simulink model "SML_SSE_RL"  (R2015a)
settings: Solver=ode4  SolverMode=MultiTasking  StartTime=0.0  StopTime=inf  FixedStep=BKIN_STEP_TIME  RelTol=1e-3
StartFcn:
  |  warndlg('Dexterit-E models cannot run under simulation. Please compile your model and run it from within Dexterit-E.');set_param(bdroot,'SimulationCommand','stop')
model workspace (MAT data in the model file):
  col_x = 1
  col_y = 2
  RADIUS_VIS = 3
  COLOR_INIT = 6
  BKIN_STEP_TIME = 0.00025
  E_END_TRIAL = 20
  STROKE_WIDTH = 8
  K_ROBOT_RAMP_TIME = 1
  E_ENABLED_CONTROLLER = 31
  K_TIME_TO_START = 4
  BKIN_KINEMATIC_FRAME_SIZE = 400
  E_NO_EVENT = 0
  STARTTARGET_COL = 1
  MOVE_TIME_COL = 3
  MOVE_XVEL_COL = 4
  MOVE_YVEL_COL = 5
  E_INIT_TRIAL = 1
  E_MOVE_TO_START = 2
  E_AT_START = 4
  E_PASSIVE_HOLD_AT_START = 6
  E_MOVE_TO_END = 8
  COLOR_SELECT = 7
  ACTORPAS_COL = 6
  E_ACTIVE_HOLD_AT_START = 7
  CHANNEL_WIDTH = 1
  WALL_WIDTH = 2
  WALL_STIFFNESS = 3
  WALL_VISCOSITY = 4
  PROBE_COL = 8
  K_TIME_HOLD_START = 5
  E_ENABLE_BUTTONS = 46
  E_DISABLE_BUTTONS = 47
  LABEL_1 = 3
  RESPONSE_AHEAD = 4
  RESPONSE_BEHIND = 5
  B_LABEL_1 = 3
  B_AHEAD = 4
  B_BEHIND = 5
  DYNOREND_COL = 7
  E_REPEAT_TRIAL_FLAG = 35
  END_TARGET_COL = 2
  HEIGHT_VIS = 4
  WIDTH_VIS = 5
  E_TOO_FAST = 11
  E_TOO_SLOW = 12
  PROBE_SHIFT_COL = 9
  K_TIME_PROBE_HOLD = 3
  E_AT_END_TARGET = 10
  K_DELAY_POSTTRIAL = 2
  LABEL_TEXT = 9
  LABEL_HEIGHT = 10
  E_FINISH_MOVE = 49
  E_HIT_PROBE = 48
  E_TEST_1 = 50
  E_JUST_RIGHT = 51
undefined symbols (not defined in the file): slselsubs
libraries: slrtlib x5, KINARM_loads x4, Video x4, General x3, KINARM_general x2, simulink x1, xpcnilib x1
(part 1 of 2)
CloseFcn:
  | rtwprivate ssgencode ModelCloseRequest b2lab2d
settings Model: ModifiedComment=chris -- Wed Feb 16 09:18:30 2005 -- Version 1.1384  ModifiedHistory=Feb 16/05 - Add error repeat, add offset ramp  ExtModeArmWhenConnect=off  ExtModeLogAll=off  Creator=Chris Grebeldinger  LastModifiedBy=User
settings SolverCC: EnableConcurrentExecution=on  AutoInsertRateTranBlk=on
settings DataIOCC: LimitDataPoints=off  SignalLoggingSaveFormat=ModelDataLogs  SaveOutput=off  SaveTime=off  SignalLoggingName=sigsOut
settings OptimizationCC: BlockReduction=off  BooleanDataType=off  OptimizeBlockIOStorage=off  BufferReuse=off  GlobalBufferReuse=off  ExpressionFolding=off  ExpressionDepthLimit=2147483647  LocalBlockOutputs=off  InitFltsAndDblsToZero=on
settings DebuggingCC: SaveWithParameterizedLinksMsg=none  UnderspecifiedInitializationDetection=Classic  MergeDetectMultiDrivingBlocksExec=none  SignalResolutionControl=TryResolveAllWithWarning  MultiTaskDSMMsg=warning  FcnCallInpInsideContextMsg=UseLocalSettings  StateNameClashWarn=warning  StrictBusMsg=ErrorOnBusTreatedAsVector
settings HardwareCC: ProdIntDivRoundTo=Zero  ProdEndianess=LittleEndian  ProdLongLongMode=on  ProdHWDeviceType=Generic->32-bit x86 compatible  TargetHWDeviceType=32-bit Generic
settings SFSimCC: SimCustomHeaderCode="#include \"stdlib.h\""  SFSimEcho=off  SimParseCustomCode=off
settings RTWCC: SystemTargetFile=slrt.tlc  TemplateMakefile=slrt_default_tmf  Description=Simulink Real-Time  CustomSourceCode="#include \"stdlib.h\""
settings CodeAppCC: MaxIdLength=63
settings SimulinkRealTimeCC: TargetFcnLib=ansi_tfl_tmw.mat  GeneratePreprocessorConditionals=Disable all  xPCisDownloadable=off  xPCisDefaultEnv=off

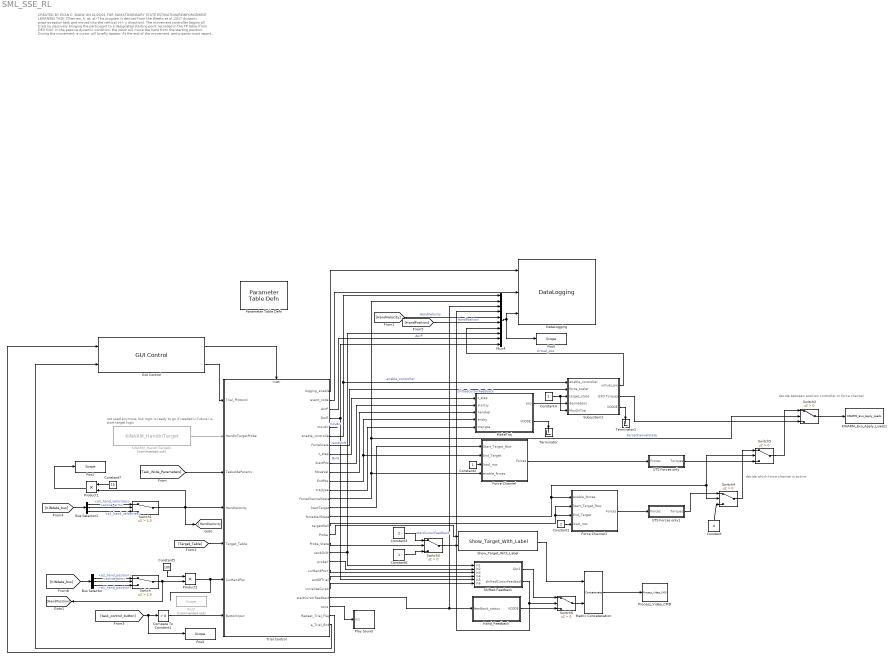
== system SML_SSE_RL ==
  note: not used anymore, but logic is ready to go if needed in future
      | i.e. start target logic
  note: decide between position controller or force channel
  note: decide which force channel is active
  note: CREATED BY EVAN C. SNOW ON 01/25/21 FOR SOMATOSENSORY STATE ESTIMATION/REINFORCEMENT LEARNING TASK (Therrien, A. et. al)
      | This program is derived from the Weeks et al. 2017 dynamic proprioception task and moved into the vertical (+/- y direction). The movement controller begins all trials by passively bringing the participant to a designated starting point recorded in the TP table (from DEX GUI).
      |
      | In the passive dynamic condition, the robot will move the hand from the starting position. During the movement, a cursor will briefly appear. At the end of the movement, participants must report if the cursor was "ahead" or "behind".
      |
      | In the passive endpoint condition, the robot will move the hand from the starting position to a designated probe somewhere between the start and end points (designated by the TP table in DEX GUI). It will then hold the fingertip veridical to the center of the probe and briefly display a cursor. After extinguishing the cursor, the movement controller will move the finger tip from the probe to the end target. At the end of the movement, participants must report if the cursor was "ahead" or "behind".
      |
      | In the active dynamic condition, participants will be held at a start point until a beep sounds, then they begin moving (as instructed). A cursor will appear briefly during the movement. The robot will stop the participant's hand at the end point. The participant must then report if the cursor was "ahead" or "behind". A force channel will enforce movement direction, and behavioral feedback will be used to maintain movement speed.
      |
      | In the active endpoint condition, participants will be held at a start point until a beep sounds, then they begin moving (as instructed). A cursor will appear briefly during the movement. The robot will stop the participant's hand at the y location of the probe and a cursor will briefly display. After extinguishing the cursor, the participant will move the finger tip from the probe to the end target. The participant must then report if the cursor was "ahead" or "behind". A force channel will enforce movement direction, and behavioral feedback will be used to maintain movement speed (behavioral feedback for this section is based on both phases individually i.e. start to probe and probe to end).
      |
      | For all trials, the cursor could be shifted +/- 0, 7, 13, 20, 30, 40 mm. The movement controller constant velocity was set to 0.5 m/s. The cursor was shown veridically before movement for 600 ms and somewhere between the start and endpoint (probe location) for 600 ms with logic depending on each task. The recording of the response from the patient is recorded using Task Buttons and is evident in the DEX GUI.
  Bus Selector : BusSelector  OutputSignals=Robot2.a2_hand_position,KINDataGeneral.active_arm,Robot1.a1_hand_position
  Bus Selector1 : BusSelector  OutputSignals=Robot2.a2_hand_velocities,KINDataGeneral.active_arm,Robot1.a1_hand_velocities
  Compare To Constant1 : simulink/Logic and Bit Operations/Compare To Constant  relop=>  const=0  OutDataTypeStr=boolean
  Constant : Constant  Value=0
  Constant1 : Constant  Value=2
  Constant2 : Constant
  Constant3 : Constant  Value=2
  Constant4 : Constant
  Constant5 : Constant  Value=100
  Constant6 : Constant
  Constant7 : Constant  Value=10
  DataLogging : General/DataLogging  log_event_codes=on  log_analog_inputs=on  show_time_remaining=off  ecat_include=on
  Force Channel : Subsystem
  Force Channel1 : Subsystem
  GUI Control : General/GUI Control  task_version=1.0  show_repeat_trial_flag=on  use_custom_tp=off  target_type_str=Circle  Target_Type=1  XYcols=[1 2]  Vcols=3  Lcols=4  indices_padding=[0 0 0 0;0 0 0 0]  target_table_rows=64  load_table_rows=20  tp_table_rows=100
  Hand_Feedback : Subsystem  AncestorBlock=KINARM_general/Hand_Feedback  mask(Hand_Feedback){feedback_cntl_src=status only}
      mask prompts: feedback_cntl_src "Task Program control of style and status"
      mask help:
      | This block controls various options for hand feedback (i.e. fingertip position)  to be shown to the subject.
      |
      | Task Program control of style and status refers to whether the Program Task will explicity control the style and/or status of the hand feedback.
      mask init:
      | block_path = gcb;  % store block path, as gcb may change with block operations
      | 
      | %%% Handle background colours if link status changes.  
      | checkBackgroundColour(block_path, 'KINARM_general');
      | 
      | 
      | feedback_cntl_source=get_param(gcb,'feedback_cntl_src');
      | 
      | if feedback_cntl_source(1:4)=='none'
      |     block1type='Constant';
      |     block2type='Constant';
      |     block3type='Constant';
      | elseif feedback_cntl_source(1:4)=='stat'
      |     block1type='Constant';
      |     block2type='Constant';
      |     block3type='Inport';
      | else 
      |     block1type='Inport';
      |     block2type='Inport';
      |     block3type='Constant';
      | end
      | 
      | hasOldName1 = ~isempty(find_system(gcb, 'FollowLinks', 'on', 'LookUnderMasks', 'all', 'name', 'Dom_VCODE'));
      | hasOldName2 = ~isempty(find_system(gcb, 'FollowLinks', 'on', 'LookUnderMasks', 'all', 'name', 'non-Dom_VCODE'));
      | 
      | block1name='Assess_arm_VCODE';
      | block2name='Contralateral_arm_VCODE';
      | block1path=[gcb '/' block1name];
      | block2path=[gcb '/' block2name];
      | 
      | if hasOldName1
      | 	set_param([gcb '/Dom_VCODE'],'name', block1name);
      | end
      | 
      | if hasOldName2
      | 	set_param([gcb '/non-Dom_VCODE'],'name', block2name);
      | end
      | 
      | if ~strcmp(get_param(block1path,'blocktype'),block1type)
      | 	pos=get_param(block1path,'position');
      | 	delete_line(gcb, [block1name '/1'], 'Reshape/1');
      | 	delete_block(block1path);
      | 	add_block(['built-in/' block1type], block1path,'Name',block1name);
      | 	set_param(block1path,'position',pos);
      | 	add_line(gcb, [block1name '/1'], 'Reshape/1');
      | end
      | 
      | if ~strcmp(get_param(block2path,'blocktype'),block2type)
      | 	pos=get_param(block2path,'position');
      | 	delete_line(gcb, [block2name '/1'], 'Reshape1/1');
      | 	delete_block(block2path);
      | 	add_block(['built-in/' block2type],block2path,'Name',block2name);
      | 	set_param(block2path,'position',pos);
      | 	add_line(gcb, [block2name '/1'], 'Reshape1/1');
      | end
      | 
      | block3name='feedback_status';
      | block3path=[gcb '/' block3name];
      | if ~strcmp(get_param(block3path,'blocktype'),block3type)
      | 	pos=get_param(block3path,'position');
      | 	delete_line(gcb, [block3name '/1'], 'FeedFwdArm/3');
      | 	delete_block(block3path);
      | 	add_block(['built-in/' block3type],block3path,'Name',block3name);
      | 	set_param(block3path,'position',pos);
      | 	add_line(gcb, [block3name '/1'], 'FeedFwdArm/3');
      | end
      | 
      | if feedback_cntl_source(1:4)=='none'
      | 	set_param(block1path,'Value','[1:70]');
      | 	set_param(block2path,'Value','[71:140]');
      | elseif feedback_cntl_source(1:4)=='stat'
      | 	set_param(block1path,'Value','[1:70]');
      | 	set_param(block2path,'Value','[71:140]');
      | end
      mask Help:
      | Creates VCODE for drawing hand position (fingertip).
      | <P>
      | <H2>Library </H2>
      | KINARM general
      | 
      | <H2>Description </H2>
      | This block controls various options for drawing hand feedback.  (Note: although it is called hand feedback, it is actually the fingertip position that is shown).  Three options are available (as chosen in the Parameters and Dialog box):
      | <P>
      | (i) GUI control of feedback style and status
      | <Blockquote>
      | No inputs are required for this option.  The Task Program has no control over the style or status of the hand feedback.
      | </Blockquote>
      | (ii) Task Program control of feedback status and GUI control of style
      | <Blockquote>
      | If Task Program control of feedback status is chosen, then one input appears for this block:<P>
      | <B> feedback_status: </B> this scalar input dynamically controls the status of the hand feedback as per the following:
      | <P>
      | 0 = (no hand feedback)<BR>
      | 1 = ("arm to be assessed" hand feedback only)<BR>
      | 2 = (contralateral arm hand feedback only)<BR>
      | 3 = (hand feedback on for both hands)<BR>
      | </Blockquote>
      | (iii) Task Program control of both feedback style and status.
      | <Blockquote>
      | 
      | If Task Program control of feedback status and style is chosen, then two inputs appear for this block:<P>
      | <B> Assess_arm_VCODE: </B>  this vector input dynamically controls the status and style of the hand feedback for the "arm to be assessed" the operator selected in Dexterit-E.
      | <P>
      | <B> Contralateral_arm_VCODE:</B>  this vector input dynamically controls the status and style of the hand feedback for the contralateral hand.
      | <P>
      | For both the Assess_arm_VCODE and the Contralateral_arm_VCODE, the input vectors must be in the appropriate VCODE format (for more information on the details of a VCODE, please right click on the Show_Target block in the video library, "Look Under Mask" and open the Embedded Matlab function).  Note that the position information in the Dom_VCODE and non-Dom_VCODE are overwritten in this block, but all other aspects of the VCODE are passed through to the output.
      | </Blockquote>
      | Note that if Task Program control is chosen for either hand feedback status or style, the GUI will still override these settings if the Task Protocol specifies that it should do so.
      | <P>
      | There is one output from this block:
      | <P>
      | <B> VCODE: </B> this output is 2-row matrix containing 2 VCODEs.  The first VCODE is for the dominant hand feedback and the second VCODE is for the non-dominant hand feedback.  This output must go to the Process_Video_CMD block of the video library for the hand feedback to actually be shown (if any other visual targets are to be displayed, then this VCODE output must be concatenated with the other VCODES prior to connection to the Process_Video_CMD block - see Help for the Process_Video_CMD block for more information).
      | <H2>Parameters and Dialog Box</H2>
      | <B>Task Program control of style and status</B> refers to whether the Program Task will explicity control the style and/or status of the hand feedback.  The three options are: none, status only, or status and style.
      | <P>
      |  - Choosing none means that style and status are always controlled by the GUI.
      | <P>
      |  - Choosing status only means that the GUI always controls the hand feedback style, but also will create an input to this block allowing the end user to control the status dynamically.  Allowable input values are: 0 (no hand feedback), 1 (dominant hand feedback only), 2 (non-dominant hand feedback only) or 3 (hand feedback on for both hands)
      |  <P>
      | - Choosing status and style means that both the hand feedback status and style can be controlled dynamically by the Task Program.  If this option is selected, then two inputs will be created for this block: dominant VCODE and non-dominant VCODE.  These two inputs require a proper VCODE (e.g. from a Show_Target block) for each.  Because status and style are both part of a VCODE, there is no separate input for hand feedback status.  Note: any position information of these input VCODEs is overwritten by this block by the appropriate fingertip locations.
      | <P>
      | 
      | <H2>Related Blocks </H2>
      | DataLogging<BR>
      | Show_Target<BR>
      | Process_Video_CMD
      mask TypeOptions feedback_cntl_src: none | status only | style and status
  KINARM_Exo_Apply_Loads1 : KINARM_loads/KINARM_Exo_Apply_Loads  up_duration=200  down_duration=200  max_torque=12  limit_motors=off
  KINARM_HandInTarget1 : KINARM_general/KINARM_HandInTarget  Commented=on  use_dominant_hand=on  target_type=Rectangle  num_states=1  attribcol1=[5 4 0]  attribcol2=[0 0 0]  attribcol3=[0 0 0]  attribcol4=[0 0 0]  attribcol5=[0 0 0]
  MakeTraj : Subsystem
  Matrix Concatenation : Concatenate  Mode=Multidimensional array
  Mux4 : Mux  Inputs=10
  Parameter Table Defn : General/Parameter Table Defn  ShowInLibBrowser=0
  Play Sound : Subsystem
  Pos1 : slrtlib/Displays and Logging/Scope   scopeno=4  scopetype=Target  autostart=on  viewmode=Graphical redraw  formatstr='%15.6f'  grid=on  ylimits=[-1,1]  nosamples=250  noprepostsamples=0  interleave=1  triggermode=FreeRun  triggersignal=1  trigsignalfromport=off  triggerlevel=0.0  triggerslope=Either  triggerscope=1  triggersample=0  filename=data.dat  mode=Lazy  writesize=512  autorestart=off  dynamicfilemode=off  maxwritefilesize=512*1024^2
  Pos2 : slrtlib/Displays and Logging/Scope   Commented=on  scopeno=3  scopetype=Target  autostart=on  viewmode=Numerical  formatstr='%15.6f'  grid=on  ylimits=[-10,10]  nosamples=250  noprepostsamples=0  interleave=1  triggermode=FreeRun  triggersignal=1  trigsignalfromport=off  triggerlevel=0.0  triggerslope=Either  triggerscope=1  triggersample=0  filename=data.dat  mode=Lazy  writesize=512  autorestart=off  dynamicfilemode=off  maxwritefilesize=512*1024^2
  Pos3 : slrtlib/Displays and Logging/Scope   scopeno=5  scopetype=Target  autostart=on  viewmode=Numerical  formatstr='%15.6f'  grid=on  ylimits=[-10,10]  nosamples=250  noprepostsamples=0  interleave=1  triggermode=FreeRun  triggersignal=1  trigsignalfromport=off  triggerlevel=0.0  triggerslope=Either  triggerscope=1  triggersample=0  filename=data.dat  mode=Lazy  writesize=512  autorestart=off  dynamicfilemode=off  maxwritefilesize=512*1024^2
  Pos5 : slrtlib/Displays and Logging/Scope   scopeno=1  scopetype=Target  autostart=on  viewmode=Numerical  formatstr='%15.6f'  grid=on  ylimits=[-10,10]  nosamples=250  noprepostsamples=0  interleave=1  triggermode=FreeRun  triggersignal=1  trigsignalfromport=off  triggerlevel=0.0  triggerslope=Either  triggerscope=1  triggersample=0  filename=data.dat  mode=Lazy  writesize=512  autorestart=off  dynamicfilemode=off  maxwritefilesize=512*1024^2
  Process_Video_CMD : Video/Process_Video_CMD  video_delay=50
  Product1 : Product
  Product2 : Product
  "Shifted Feedback " : Subsystem
  Show_Target_With_Label : Video/Show_Target_With_Label  target_type=Circle  num_states=2  attribcol1=[0 0 0 0 0 0 0]  attribcol2=[0 0 0 0 LABEL_TEXT COLOR_SELECT LABEL_HEIGHT]  attribcol3=[0 0 0 0 0 0 0]  attribcol4=[0 0 0 0 0 0 0]  attribcol5=[0 0 0 0 0 0 0]  stateindices_padding=[0 0 0 0;0 0 0 0;0 0 0 0;0 0 0 0;0 0 0 0]  source=dialog  opacity=100  target_display=Both subject and operator displays
  Subsystem2 : Subsystem
  Switch : Switch  Criteria=u2 > Threshold  Threshold=1.5
  Switch1 : Switch  Criteria=u2 > Threshold  Threshold=1.5
  Switch{2..6} (5 alike) : Switch  Criteria=u2 > Threshold
  Terminator : Terminator
  Terminator1 : Terminator
  Trial Control : Stateflow chart  TreatAsAtomicUnit=on
  UTS Forces only : Subsystem
  UTS Forces only1 : Subsystem
  wires:
  [Task_Wide_Parameters] -> Trial Control/3(TaskwideParams)
  Trial Control/2(event_code) -> DataLogging/2
  Switch1/1 -> Product1/2, [HandVelocity], Trial Control/4(HandVelocity)
  Bus Selector1/3 -> Switch1/3  "<a1_hand_velocities>"
  Bus Selector1/1 -> Switch1/1  "<a2_hand_velocities>"
  [KINdata_bus] -> Bus Selector1/1
  GUI Control/2 -> Trial Control/1(Trial_Protocol)
  Trial Control/8(t_step) -> MakeTraj/1(t_step)
  Trial Control/25(tone) -> Play Sound/1(In1)
  [Target_Table] -> Trial Control/5(Target_Table)
  Trial Control/26(Repeat_Trial_Flag) -> GUI Control/1
  GUI Control/1 -> Trial Control/Trigger
  Mux4/1 -> Pos5/1, DataLogging/3
  Trial Control/1(logging_enable) -> DataLogging/1
  Subsystem2/2(EXO Torques) -> Switch2/3
  Trial Control/27(e_Trial_End) -> GUI Control/2
  MakeTraj/1(pos) -> Subsystem2/4(desiredpos)
  Subsystem2/1(virtual_pos) -> Mux4/7  "virtual_pos"
  Constant4/1 -> Subsystem2/5(MovOnTraj), Subsystem2/3(target_state)
  Trial Control/6(enable_controller) -> Mux4/1, Subsystem2/1(enable_controller)  "enable_controller"
  [KINdata_bus] -> Bus Selector/1
  Bus Selector/2 -> Switch/2  "<active_arm>"
  Bus Selector/1 -> Switch/1  "<a2_hand_position>"
  Bus Selector/3 -> Switch/3  "<a1_hand_position>"
  Switch/1 -> [HandPosition], Product2/2
  Constant5/1 -> Product2/1
  Product2/1 -> Trial Control/6(CurHandPos)
  Matrix Concatenation/1 -> Process_Video_CMD/1
  Trial Control/9(StartPos) -> MakeTraj/2(startxy)
  Trial Control/10(MoveVel) -> MakeTraj/3(handvel)
  Trial Control/11(EndPos) -> MakeTraj/4(endxy), Force Channel/2(End_Target)
  Trial Control/12(trajtype) -> MakeTraj/5(trajtype)
  Trial Control/3(AorP) -> Mux4/9  "AorP"
  Force Channel/1(Forces) -> UTS Forces only/1(Forces)
  Trial Control/7(ForceScale) -> Subsystem2/2(force_scaler)
  Bus Selector1/2 -> Switch1/2  "<active_arm>"
  Trial Control/14(StartTarget) -> Force Channel/1(Start_Target_Row)
  Constant2/1 -> Force Channel/3(load_row)
  Trial Control/13(ForceChannelState) -> Mux4/2, Switch2/2, Force Channel/4(enable_forces)  "ForceChannelState"
  Switch2/1 -> KINARM_Exo_Apply_Loads1/1
  MakeTraj/2(VCODE) -> Terminator/1
  Subsystem2/3(VCODE) -> Terminator1/1
  Trial Control/17(Probe) -> Show_Target_With_Label/1
  KINARM_HandInTarget1/1 -> Trial Control/2(HandInTargetProbe)
  Trial Control/18(Probe_State) -> Switch3/2
  Constant3/1 -> Switch3/1
  Constant6/1 -> Switch3/3
  Switch3/1 -> Show_Target_With_Label/2
  Show_Target_With_Label/1 -> Matrix Concatenation/1
  Compare To Constant1/1 -> Trial Control/7(ButtonInput)
  Trial Control/19(randShift) -> Mux4/8, "Shifted Feedback "/1(In1)  "randShift"
  Trial Control/20(probeY) -> "Shifted Feedback "/2(In2)
  Trial Control/21(curHandPosY) -> "Shifted Feedback "/3(In3)
  Trial Control/22(endOfTrial) -> "Shifted Feedback "/4(In4)
  Hand_Feedback/1(VCODE) -> Switch6/3
  Trial Control/24(startCursorFeedback) -> Mux4/3, Hand_Feedback/1(feedback_status)  "startCursorFeedback"
  Trial Control/5(movdir) -> ?  "movdir"
  Switch4/1 -> Switch5/1
  Constant/1 -> Switch4/3
  Trial Control/15(forceWallState) -> Force Channel1/1(enable_forces), Switch4/2, Switch5/2
  Constant1/1 -> Force Channel1/4(load_row)
  Force Channel1/1(Forces) -> UTS Forces only1/1(Forces)
  UTS Forces only1/1(Torques) -> Switch4/1
  Trial Control/16(targetWall) -> Force Channel1/2(Start_Target_Row), Force Channel1/3(End_Target)
  UTS Forces only/1(Torques) -> Switch5/3
  Switch5/1 -> Switch2/1
  Trial Control/4(DorE) -> Mux4/10, "Shifted Feedback "/5(In5)  "DorE"
  "Shifted Feedback "/1(Out1) -> Switch6/1
  "Shifted Feedback "/2(shiftedCursorFeedback) -> Mux4/4, Switch6/2  "shiftedCursorFeedback"
  Switch6/1 -> Matrix Concatenation/2
  Trial Control/23(initializeCursor) -> "Shifted Feedback "/6(In6)
  [HandVelocity] -> Mux4/5  "HandVelocity"
  Constant7/1 -> Product1/1
  Product1/1 -> Pos1/1
  [task_control_button] -> Pos3/1, Compare To Constant1/1
  [HandPosition] -> Mux4/6  "HandPosition"

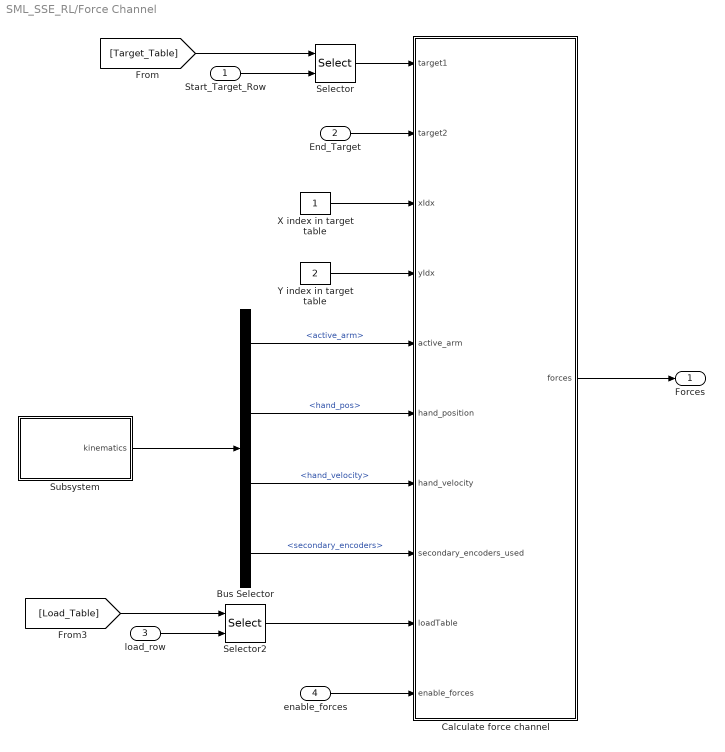
== system SML_SSE_RL/Force Channel ==
  Start_Target_Row : Inport
  End_Target : Inport  Port=2
  load_row : Inport  Port=3
  enable_forces : Inport  Port=4
  Bus Selector : BusSelector  OutputSignals=active_arm,hand_pos,hand_velocity,secondary_encoders
  Calculate force channel : MATLAB Function  TreatAsAtomicUnit=on
  Selector : Selector  NumberOfDimensions=2  InputPortWidth=3  IndexOptions=Index vector (port),Select all  Indices=1,-1  OutputSizes=slselsubs([(-2),(-2)],1),slselsubs([(-2),(-2)],2)
  Selector2 : Selector  NumberOfDimensions=2  InputPortWidth=3  IndexOptions=Index vector (port),Select all  Indices=1,-1  OutputSizes=slselsubs([(-2),(-2)],1),slselsubs([(-2),(-2)],2)
  Subsystem : Subsystem
  X index in target table : Constant
  Y index in target table : Constant  Value=2
  Forces : Outport
  wires:
  Selector/1 -> Calculate force channel/1(target1)
  [Target_Table] -> Selector/1
  Start_Target_Row/1 -> Selector/2
  End_Target/1 -> Calculate force channel/2(target2)
  X index in target table/1 -> Calculate force channel/3(xIdx)
  Y index in target table/1 -> Calculate force channel/4(yIdx)
  enable_forces/1 -> Calculate force channel/10(enable_forces)
  [Load_Table] -> Selector2/1
  load_row/1 -> Selector2/2
  Selector2/1 -> Calculate force channel/9(loadTable)
  Calculate force channel/1(forces) -> Forces/1
  Subsystem/1(kinematics) -> Bus Selector/1
  Bus Selector/1 -> Calculate force channel/5(active_arm)  "<active_arm>"
  Bus Selector/2 -> Calculate force channel/6(hand_position)  "<hand_pos>"
  Bus Selector/3 -> Calculate force channel/7(hand_velocity)  "<hand_velocity>"
  Bus Selector/4 -> Calculate force channel/8(secondary_encoders_used)  "<secondary_encoders>"

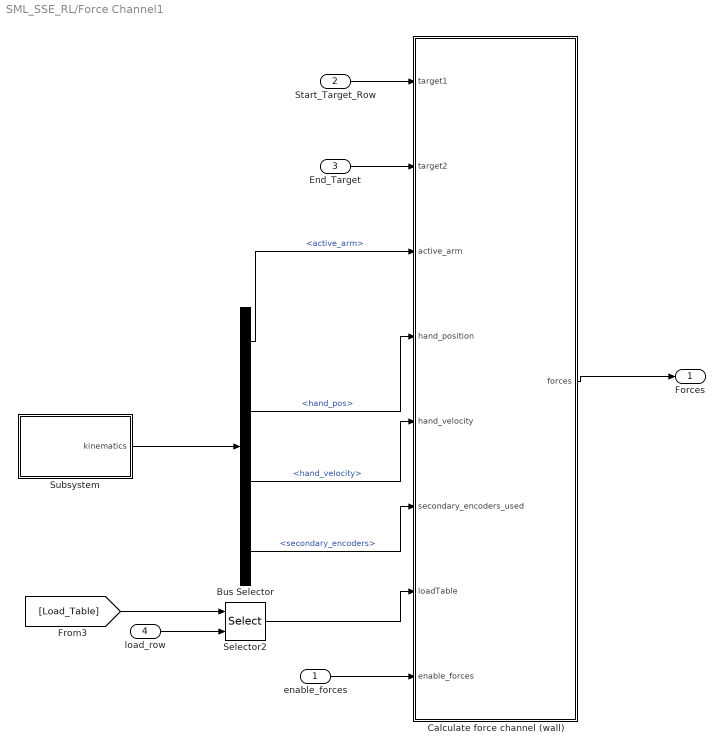
== system SML_SSE_RL/Force Channel1 ==
  enable_forces : Inport
  Start_Target_Row : Inport  Port=2
  End_Target : Inport  Port=3
  load_row : Inport  Port=4
  Bus Selector : BusSelector  OutputSignals=active_arm,hand_pos,hand_velocity,secondary_encoders
  "Calculate force channel (wall) " : MATLAB Function  TreatAsAtomicUnit=on
  Selector2 : Selector  NumberOfDimensions=2  InputPortWidth=3  IndexOptions=Index vector (port),Select all  Indices=1,-1  OutputSizes=slselsubs([(-2),(-2)],1),slselsubs([(-2),(-2)],2)
  Subsystem : Subsystem
  Forces : Outport
  wires:
  Bus Selector/4 -> "Calculate force channel (wall) "/6(secondary_encoders_used)  "<secondary_encoders>"
  Bus Selector/3 -> "Calculate force channel (wall) "/5(hand_velocity)  "<hand_velocity>"
  Bus Selector/2 -> "Calculate force channel (wall) "/4(hand_position)  "<hand_pos>"
  Bus Selector/1 -> "Calculate force channel (wall) "/3(active_arm)  "<active_arm>"
  Subsystem/1(kinematics) -> Bus Selector/1
  "Calculate force channel (wall) "/1(forces) -> Forces/1
  Selector2/1 -> "Calculate force channel (wall) "/7(loadTable)
  load_row/1 -> Selector2/2
  [Load_Table] -> Selector2/1
  enable_forces/1 -> "Calculate force channel (wall) "/8(enable_forces)
  End_Target/1 -> "Calculate force channel (wall) "/2(target2)
  Start_Target_Row/1 -> "Calculate force channel (wall) "/1(target1)

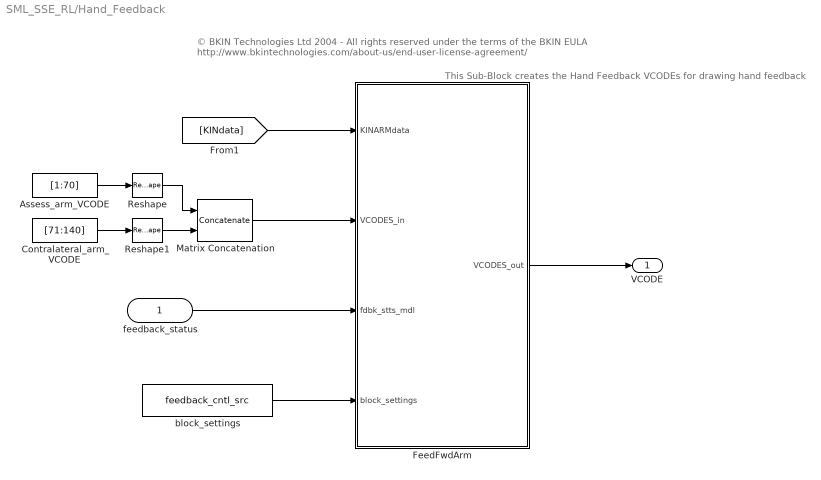
== system SML_SSE_RL/Hand_Feedback ==
  note: This Sub-Block creates the Hand Feedback VCODEs for drawing hand feedback
  note: © BKIN Technologies Ltd 2004  - All rights reserved under the terms of the BKIN EULA
      | http://www.bkintechnologies.com/about-us/end-user-license-agreement/
  feedback_status : Inport
  Assess_arm_VCODE : Constant  Value=[1:70]
  Contralateral_arm_VCODE : Constant  Value=[71:140]
  FeedFwdArm : MATLAB Function  TreatAsAtomicUnit=on
      settings: RTWSystemCode=Nonreusable function  RTWFileNameOpts=Use function name
  Matrix Concatenation : Concatenate  Mode=Multidimensional array
  Reshape : Reshape  OutputDimensionality=Row vector (2-D)
  Reshape1 : Reshape  OutputDimensionality=Row vector (2-D)
  block_settings : Constant  Value=feedback_cntl_src
  VCODE : Outport
  wires:
  Contralateral_arm_VCODE/1 -> Reshape1/1
  Assess_arm_VCODE/1 -> Reshape/1
  FeedFwdArm/1(VCODES_out) -> VCODE/1
  block_settings/1 -> FeedFwdArm/4(block_settings)
  Matrix Concatenation/1 -> FeedFwdArm/2(VCODES_in)
  [KINdata] -> FeedFwdArm/1(KINARMdata)
  Reshape1/1 -> Matrix Concatenation/2
  Reshape/1 -> Matrix Concatenation/1
  feedback_status/1 -> FeedFwdArm/3(fdbk_stts_mdl)

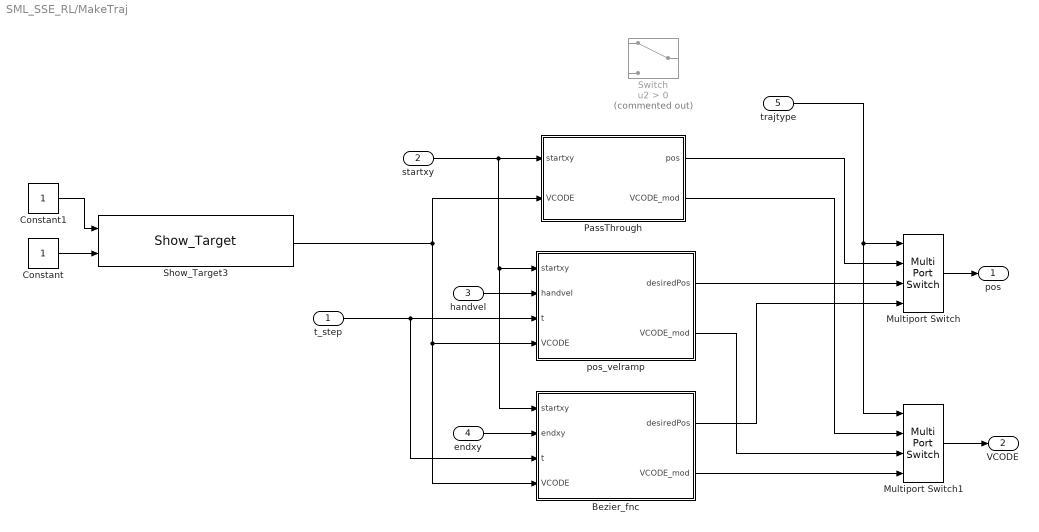
== system SML_SSE_RL/MakeTraj ==
  t_step : Inport  PortDimensions=1
  startxy : Inport  Port=2  PortDimensions=[1 2]
  handvel : Inport  Port=3
  endxy : Inport  Port=4
  trajtype : Inport  Port=5  PortDimensions=1
  Bezier_fnc : MATLAB Function  TreatAsAtomicUnit=on
  Constant : Constant
  Constant1 : Constant
  Multiport Switch : MultiPortSwitch  DataPortOrder=Specify indices  DataPortIndices={2,1,0}  DiagnosticForDefault=Warning
  Multiport Switch1 : MultiPortSwitch  DataPortOrder=Specify indices  DataPortIndices={2,1,0}  DiagnosticForDefault=Warning
  PassThrough : MATLAB Function  TreatAsAtomicUnit=on
  Show_Target3 : Video/Show_Target  target_type=Circle  num_states=1  attribcol1=[COLOR_INIT 0 0 RADIUS_VIS]  attribcol2=[0 0 0 0]  attribcol3=[0 0 0 0]  attribcol4=[0 0 0 0]  attribcol5=[0 0 0 0]  stateindices_padding=[0 0 0 0 0 0 0;0 0 0 0 0 0 0;0 0 0 0 0 0 0;0 0 0 0 0 0 0;0 0 0 0 0 0 0]  source=dialog  opacity=100  target_display=Both subject and operator displays  num_col=4
  Switch : Switch  Commented=on  Criteria=u2 > Threshold
  pos_velramp : MATLAB Function  TreatAsAtomicUnit=on
  pos : Outport  OutDataTypeStr=double  PortDimensions=[1 2]
  VCODE : Outport  Port=2
  wires:
  Show_Target3/1 -> Bezier_fnc/4(VCODE), pos_velramp/4(VCODE), PassThrough/2(VCODE)
  Constant1/1 -> Show_Target3/1
  startxy/1 -> Bezier_fnc/1(startxy), pos_velramp/1(startxy), PassThrough/1(startxy)
  Constant/1 -> Show_Target3/2
  t_step/1 -> Bezier_fnc/3(t), pos_velramp/3(t)
  handvel/1 -> pos_velramp/2(handvel)
  endxy/1 -> Bezier_fnc/2(endxy)
  Multiport Switch/1 -> pos/1
  Multiport Switch1/1 -> VCODE/1
  pos_velramp/1(desiredPos) -> Multiport Switch/3
  Bezier_fnc/1(desiredPos) -> Multiport Switch/4
  pos_velramp/2(VCODE_mod) -> Multiport Switch1/3
  Bezier_fnc/2(VCODE_mod) -> Multiport Switch1/4
  trajtype/1 -> Multiport Switch1/1, Multiport Switch/1
  PassThrough/1(pos) -> Multiport Switch/2
  PassThrough/2(VCODE_mod) -> Multiport Switch1/2

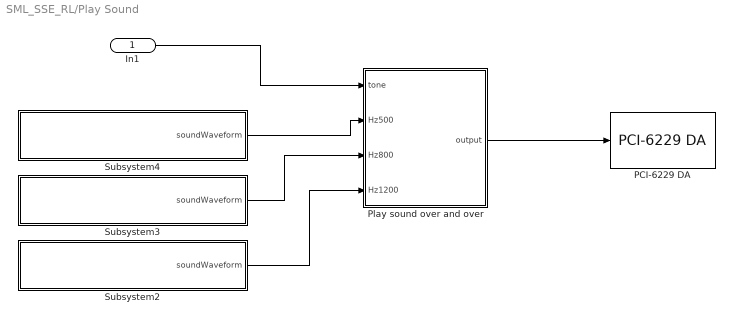
== system SML_SSE_RL/Play Sound ==
  In1 : Inport
  PCI-6229 DA : xpcnilib/D//A/M Series/PCI-6229 DA  channel=[1]  reset=[1]  initValue=[0]  sampletime=-1  slot=-1
  Play sound over and over : MATLAB Function  TreatAsAtomicUnit=on
  Subsystem2 : Subsystem  mask(Load Waveform Into Variable){fileName=Hz1200}
      mask prompts: fileName "Name of .mat Data File (must be in current directory)"
      mask help: This block will load the .MAT file specified in the dialog, and put the first variable into a GoTo called 'soundWaveform'.
      mask init:
      | filenameFromMask = get_param(gcb, 'fileName');
      | 
      | try 
      | 	dataFromFile = load(filenameFromMask);
      | 	names = fieldnames(dataFromFile);
      | 	soundDataFromFile = dataFromFile.(names{1});
      | 	display(['Sound waveform from file ''' filenameFromMask ''' loaded.']);
      | catch ME
      | 	display(ME.message)
      | end
      mask Help:
      | Enter the name a .MAT file containing a single vector or matrix. The .MAT file must be located in the current directory.
      | 
      | The first variable from the .MAT file will be put into a Goto called 'soundWaveform'.
      mask Display: disp(['Load waveform from ''' filenameFromMask ''''])
  Subsystem3 : Subsystem  mask(Load Waveform Into Variable){fileName=Hz800}
      mask prompts: fileName "Name of .mat Data File (must be in current directory)"
      mask help: This block will load the .MAT file specified in the dialog, and put the first variable into a GoTo called 'soundWaveform'.
      mask init: same as SML_SSE_RL/Play Sound/Subsystem2
      mask Help:
      | Enter the name a .MAT file containing a single vector or matrix. The .MAT file must be located in the current directory.
      | 
      | The first variable from the .MAT file will be put into a Goto called 'soundWaveform'.
      mask Display: disp(['Load waveform from ''' filenameFromMask ''''])
  Subsystem4 : Subsystem  mask(Load Waveform Into Variable){fileName=Hz500}
      mask prompts: fileName "Name of .mat Data File (must be in current directory)"
      mask help: This block will load the .MAT file specified in the dialog, and put the first variable into a GoTo called 'soundWaveform'.
      mask init: same as SML_SSE_RL/Play Sound/Subsystem2
      mask Help:
      | Enter the name a .MAT file containing a single vector or matrix. The .MAT file must be located in the current directory.
      | 
      | The first variable from the .MAT file will be put into a Goto called 'soundWaveform'.
      mask Display: disp(['Load waveform from ''' filenameFromMask ''''])
  wires:
  Play sound over and over/1(output) -> PCI-6229 DA/1
  Subsystem3/1(soundWaveform) -> Play sound over and over/3(Hz800)
  Subsystem4/1(soundWaveform) -> Play sound over and over/2(Hz500)
  In1/1 -> Play sound over and over/1(tone)
  Subsystem2/1(soundWaveform) -> Play sound over and over/4(Hz1200)

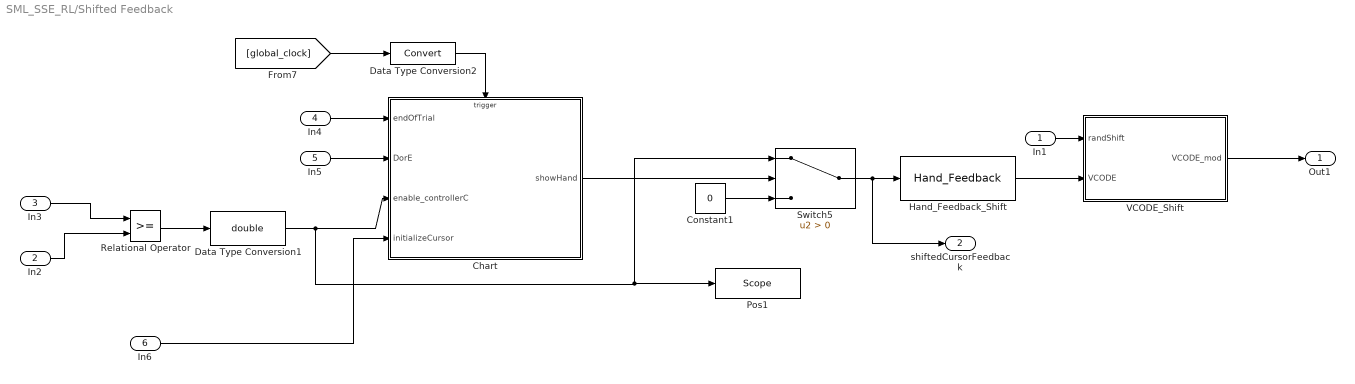
== system SML_SSE_RL/Shifted Feedback  ==
  In1 : Inport
  In2 : Inport  Port=2
  In3 : Inport  Port=3
  In4 : Inport  Port=4
  In5 : Inport  Port=5
  In6 : Inport  Port=6
  Chart : Stateflow chart  TreatAsAtomicUnit=on
  Constant1 : Constant  Value=0
  Data Type Conversion1 : DataTypeConversion  OutDataTypeStr=double  RndMeth=Round
  Data Type Conversion2 : DataTypeConversion
  "Hand_Feedback_Shift " : KINARM_general/Hand_Feedback  feedback_cntl_src=status only
  Pos1 : slrtlib/Displays and Logging/Scope   scopeno=2  scopetype=Target  autostart=on  viewmode=Numerical  formatstr='%15.6f'  grid=on  ylimits=[-10,10]  nosamples=250  noprepostsamples=0  interleave=1  triggermode=FreeRun  triggersignal=1  trigsignalfromport=off  triggerlevel=0.0  triggerslope=Either  triggerscope=1  triggersample=0  filename=data.dat  mode=Lazy  writesize=512  autorestart=off  dynamicfilemode=off  maxwritefilesize=512*1024^2
  Relational Operator : RelationalOperator  OutDataTypeStr=boolean
  Switch5 : Switch  Criteria=u2 > Threshold
  VCODE_Shift : MATLAB Function  TreatAsAtomicUnit=on
  Out1 : Outport
  shiftedCursorFeedback : Outport  Port=2
  wires:
  "Hand_Feedback_Shift "/1 -> VCODE_Shift/2(VCODE)
  VCODE_Shift/1(VCODE_mod) -> Out1/1
  Relational Operator/1 -> Data Type Conversion1/1
  Switch5/1 -> shiftedCursorFeedback/1, "Hand_Feedback_Shift "/1
  In3/1 -> Relational Operator/1
  In4/1 -> Chart/1(endOfTrial)
  Data Type Conversion1/1 -> Chart/3(enable_controllerC), Switch5/1, Pos1/1
  Constant1/1 -> Switch5/3
  Chart/1(showHand) -> Switch5/2
  In1/1 -> VCODE_Shift/1(randShift)
  [global_clock] -> Data Type Conversion2/1
  Data Type Conversion2/1 -> Chart/Trigger
  In2/1 -> Relational Operator/2
  In5/1 -> Chart/2(DorE)
  In6/1 -> Chart/4(initializeCursor)

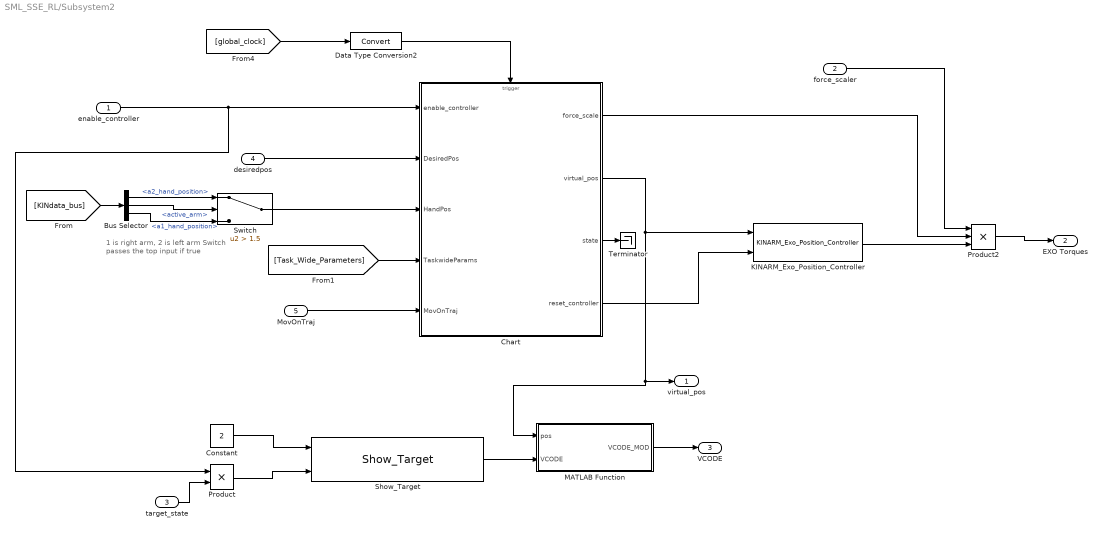
== system SML_SSE_RL/Subsystem2 ==
  note: 1 is right arm, 2 is left arm
      | Switch passes the top input if true
  enable_controller : Inport
  force_scaler : Inport  Port=2
  target_state : Inport  Port=3
  desiredpos : Inport  Port=4
  MovOnTraj : Inport  Port=5
  Bus Selector : BusSelector  OutputSignals=Robot2.a2_hand_position,KINDataGeneral.active_arm,Robot1.a1_hand_position
  Chart : Stateflow chart  TreatAsAtomicUnit=on
  Constant : Constant  Value=2
  Data Type Conversion2 : DataTypeConversion
  KINARM_Exo_Position_Controller : KINARM_loads/KINARM_Exo_Position_Controller  use_dom_hand=on  KINARM_Type=Human  inertias_for_FF=KINARM robot & arm troughs & subject  angles_or_XY=End-point (global x/y)  sample_time=0.001
  MATLAB Function : MATLAB Function  TreatAsAtomicUnit=on
  Product : Product
  Product2 : Product  Inputs=3
  Show_Target : Video/Show_Target  target_type=Circle  num_states=1  attribcol1=[COLOR_INIT 0 0 RADIUS_VIS]  attribcol2=[0 0 0 0]  attribcol3=[0 0 0 0]  attribcol4=[0 0 0 0]  attribcol5=[0 0 0 0]  stateindices_padding=[0 0 0 0 0 0 0;0 0 0 0 0 0 0;0 0 0 0 0 0 0;0 0 0 0 0 0 0;0 0 0 0 0 0 0]  source=dialog  opacity=100  target_display=Both subject and operator displays  num_col=4
  Switch : Switch  Criteria=u2 > Threshold  Threshold=1.5
  Terminator : Terminator
  virtual_pos : Outport
  EXO Torques : Outport  Port=2
  VCODE : Outport  Port=3
  wires:
  [KINdata_bus] -> Bus Selector/1
  Bus Selector/2 -> Switch/2  "<active_arm>"
  [Task_Wide_Parameters] -> Chart/4(TaskwideParams)
  [global_clock] -> Data Type Conversion2/1
  Data Type Conversion2/1 -> Chart/Trigger
  Chart/2(virtual_pos) -> MATLAB Function/1(pos), virtual_pos/1, KINARM_Exo_Position_Controller/1
  MovOnTraj/1 -> Chart/5(MovOnTraj)
  Switch/1 -> Chart/3(HandPos)
  desiredpos/1 -> Chart/2(DesiredPos)
  Constant/1 -> Show_Target/1
  Show_Target/1 -> MATLAB Function/2(VCODE)
  MATLAB Function/1(VCODE_MOD) -> VCODE/1
  KINARM_Exo_Position_Controller/1 -> Product2/3
  Product2/1 -> EXO Torques/1
  Chart/1(force_scale) -> Product2/2
  Chart/4(reset_controller) -> KINARM_Exo_Position_Controller/2
  Bus Selector/1 -> Switch/1  "<a2_hand_position>"
  Bus Selector/3 -> Switch/3  "<a1_hand_position>"
  enable_controller/1 -> Product/1, Chart/1(enable_controller)
  Product/1 -> Show_Target/2
  target_state/1 -> Product/2
  force_scaler/1 -> Product2/1
  Chart/3(state) -> Terminator/1

== system SML_SSE_RL/UTS Forces only ==
  note: Only pass through the forces if this is a UTS Exo. The
      | Classic Exo does not have the stability to control a
      | force channel well
  Forces : Inport
  Constant : Constant  Value=[0, 0, 0, 0]
  Forces_to_Torques : KINARM_loads/Forces_to_Torques
  Subsystem : Subsystem
  Switch : Switch  Criteria=u2 > Threshold
  Torques : Outport
  wires:
  Subsystem/1(isUTS) -> Switch/2
  Constant/1 -> Switch/3
  Switch/1 -> Forces_to_Torques/1
  Forces/1 -> Switch/1
  Forces_to_Torques/1 -> Torques/1

== system SML_SSE_RL/UTS Forces only1 ==
  note: Only pass through the forces if this is a UTS Exo. The
      | Classic Exo does not have the stability to control a
      | force channel well
  Forces : Inport
  Constant : Constant  Value=[0, 0, 0, 0]
  Forces_to_Torques : KINARM_loads/Forces_to_Torques
  Subsystem : Subsystem
  Switch : Switch  Criteria=u2 > Threshold
  Torques : Outport
  wires:
  Forces_to_Torques/1 -> Torques/1
  Forces/1 -> Switch/1
  Switch/1 -> Forces_to_Torques/1
  Constant/1 -> Switch/3
  Subsystem/1(isUTS) -> Switch/2

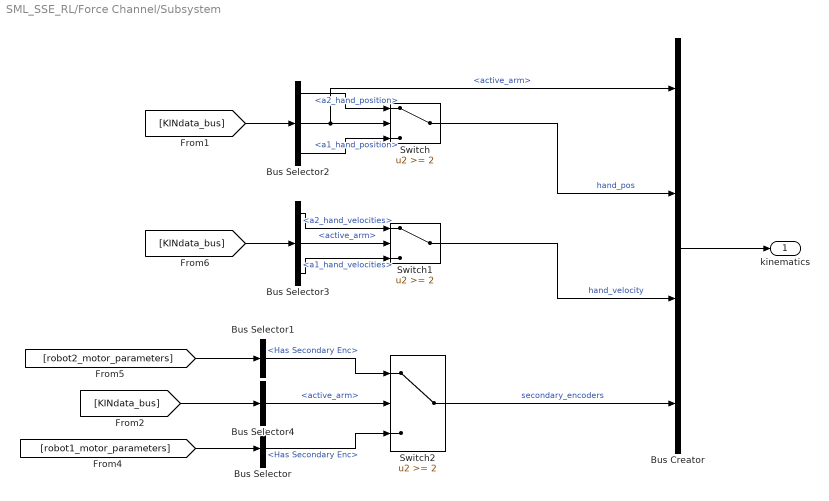
== system SML_SSE_RL/Force Channel/Subsystem ==
  Bus Creator : BusCreator
  Bus Selector : BusSelector  OutputSignals=R1.Has Secondary Enc
  Bus Selector1 : BusSelector  OutputSignals=R2.Has Secondary Enc
  Bus Selector2 : BusSelector  OutputSignals=Robot2.a2_hand_position,KINDataGeneral.active_arm,Robot1.a1_hand_position
  Bus Selector3 : BusSelector  OutputSignals=Robot2.a2_hand_velocities,KINDataGeneral.active_arm,Robot1.a1_hand_velocities
  Bus Selector4 : BusSelector  OutputSignals=KINDataGeneral.active_arm
  Switch : Switch  Threshold=2
  Switch1 : Switch  Threshold=2
  Switch2 : Switch  Threshold=2
  kinematics : Outport
  wires:
  [KINdata_bus] -> Bus Selector2/1
  Bus Selector2/1 -> Switch/1  "<a2_hand_position>"
  Bus Selector2/3 -> Switch/3  "<a1_hand_position>"
  Bus Selector2/2 -> Bus Creator/1, Switch/2  "<active_arm>"
  Bus Selector3/1 -> Switch1/1  "<a2_hand_velocities>"
  Bus Selector3/2 -> Switch1/2  "<active_arm>"
  Bus Selector3/3 -> Switch1/3  "<a1_hand_velocities>"
  [KINdata_bus] -> Bus Selector3/1
  [robot2_motor_parameters] -> Bus Selector1/1
  [robot1_motor_parameters] -> Bus Selector/1
  Bus Selector/1 -> Switch2/3  "<Has Secondary Enc>"
  Bus Selector1/1 -> Switch2/1  "<Has Secondary Enc>"
  [KINdata_bus] -> Bus Selector4/1
  Bus Selector4/1 -> Switch2/2  "<active_arm>"
  Switch/1 -> Bus Creator/2  "hand_pos"
  Switch1/1 -> Bus Creator/3  "hand_velocity"
  Switch2/1 -> Bus Creator/4  "secondary_encoders"
  Bus Creator/1 -> kinematics/1

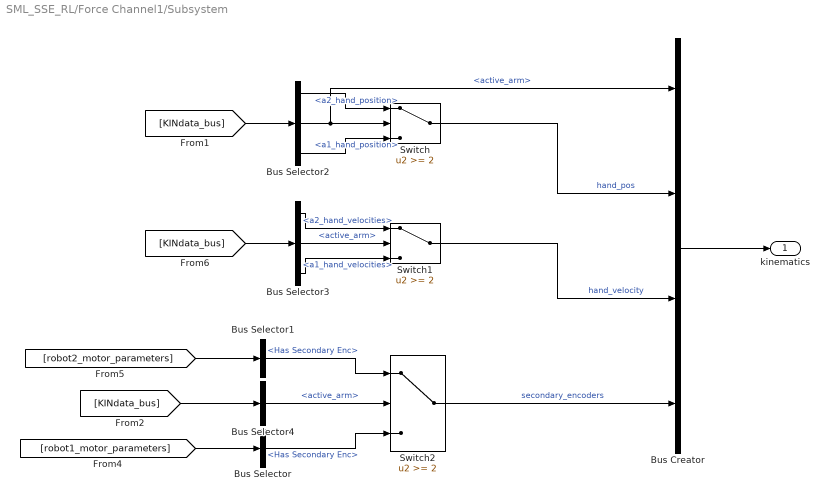
== system SML_SSE_RL/Force Channel1/Subsystem ==
  Bus Creator : BusCreator
  Bus Selector : BusSelector  OutputSignals=R1.Has Secondary Enc
  Bus Selector1 : BusSelector  OutputSignals=R2.Has Secondary Enc
  Bus Selector2 : BusSelector  OutputSignals=Robot2.a2_hand_position,KINDataGeneral.active_arm,Robot1.a1_hand_position
  Bus Selector3 : BusSelector  OutputSignals=Robot2.a2_hand_velocities,KINDataGeneral.active_arm,Robot1.a1_hand_velocities
  Bus Selector4 : BusSelector  OutputSignals=KINDataGeneral.active_arm
  Switch : Switch  Threshold=2
  Switch1 : Switch  Threshold=2
  Switch2 : Switch  Threshold=2
  kinematics : Outport
  wires:
  Bus Creator/1 -> kinematics/1
  Switch2/1 -> Bus Creator/4  "secondary_encoders"
  Switch1/1 -> Bus Creator/3  "hand_velocity"
  Switch/1 -> Bus Creator/2  "hand_pos"
  Bus Selector4/1 -> Switch2/2  "<active_arm>"
  [KINdata_bus] -> Bus Selector4/1
  Bus Selector1/1 -> Switch2/1  "<Has Secondary Enc>"
  Bus Selector/1 -> Switch2/3  "<Has Secondary Enc>"
  [robot1_motor_parameters] -> Bus Selector/1
  [robot2_motor_parameters] -> Bus Selector1/1
  [KINdata_bus] -> Bus Selector3/1
  Bus Selector3/3 -> Switch1/3  "<a1_hand_velocities>"
  Bus Selector3/2 -> Switch1/2  "<active_arm>"
  Bus Selector3/1 -> Switch1/1  "<a2_hand_velocities>"
  Bus Selector2/2 -> Switch/2, Bus Creator/1  "<active_arm>"
  Bus Selector2/3 -> Switch/3  "<a1_hand_position>"
  Bus Selector2/1 -> Switch/1  "<a2_hand_position>"
  [KINdata_bus] -> Bus Selector2/1

== system SML_SSE_RL/Play Sound/Subsystem2 ==
  Constant1 : Constant  Value=soundDataFromFile  SampleTime=-1
  soundWaveform : Outport
  wires:
  Constant1/1 -> soundWaveform/1

== system SML_SSE_RL/Play Sound/Subsystem3 ==
  Constant1 : Constant  Value=soundDataFromFile
  soundWaveform : Outport
  wires:
  Constant1/1 -> soundWaveform/1

== system SML_SSE_RL/Play Sound/Subsystem4 ==
  Constant1 : Constant  Value=soundDataFromFile
  soundWaveform : Outport
  wires:
  Constant1/1 -> soundWaveform/1

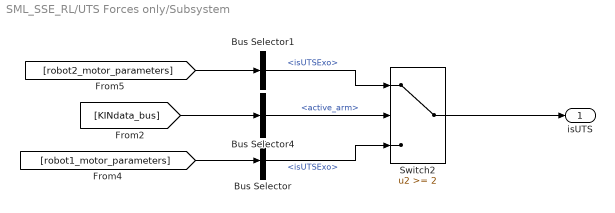
== system SML_SSE_RL/UTS Forces only/Subsystem ==
  Bus Selector : BusSelector  OutputSignals=R1Info.isUTSExo
  Bus Selector1 : BusSelector  OutputSignals=R2Info.isUTSExo
  Bus Selector4 : BusSelector  OutputSignals=KINDataGeneral.active_arm
  Switch2 : Switch  Threshold=2
  isUTS : Outport
  wires:
  [robot1_motor_parameters] -> Bus Selector/1
  Bus Selector4/1 -> Switch2/2  "<active_arm>"
  Switch2/1 -> isUTS/1
  Bus Selector1/1 -> Switch2/1  "<isUTSExo>"
  [KINdata_bus] -> Bus Selector4/1
  [robot2_motor_parameters] -> Bus Selector1/1
  Bus Selector/1 -> Switch2/3  "<isUTSExo>"

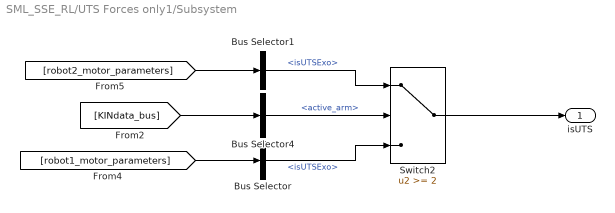
== system SML_SSE_RL/UTS Forces only1/Subsystem ==
  Bus Selector : BusSelector  OutputSignals=R1Info.isUTSExo
  Bus Selector1 : BusSelector  OutputSignals=R2Info.isUTSExo
  Bus Selector4 : BusSelector  OutputSignals=KINDataGeneral.active_arm
  Switch2 : Switch  Threshold=2
  isUTS : Outport
  wires:
  Bus Selector/1 -> Switch2/3  "<isUTSExo>"
  [robot2_motor_parameters] -> Bus Selector1/1
  [KINdata_bus] -> Bus Selector4/1
  Bus Selector1/1 -> Switch2/1  "<isUTSExo>"
  Switch2/1 -> isUTS/1
  Bus Selector4/1 -> Switch2/2  "<active_arm>"
  [robot1_motor_parameters] -> Bus Selector/1

== matlab function SML_SSE_RL/MakeTraj/Bezier_fnc ==
  data: startxy input size=[1 2]; endxy input; t input; desiredPos output size=[1 2]; VCODE input; VCODE_mod output
function [desiredPos,VCODE_mod] = fcn(startxy,endxy,t,VCODE)
%#codegen

VCODE_mod = VCODE;

%clip t just in case!
if t < 0
    t = 0;
elseif t > 1;
    t = 1;
end

t = t-sin(2*pi*t)/(2*pi);  %use the bell-shaped velocity profile from the trajectory controller

%linear bezier using origin and reference
%point from the next trial
cp1 = startxy;
cp2 = endxy;

dPos = (1-t)*cp1 + t*cp2;


desiredPos = dPos; %to get to cm
desiredPos = desiredPos/100;

VCODE_mod(3) = desiredPos(1); %convert to meters
VCODE_mod(4) = desiredPos(2); %convert to meters

== matlab function SML_SSE_RL/Shifted Feedback /VCODE_Shift ==
  data: randShift input; VCODE input; VCODE_mod output
function VCODE_mod  = fcn(randShift, VCODE)
%This function will add the shift from a set of possible shifts. For the
%time being it will be randomly generated
%randShift will be an integer 1:11

%shiftsX = [];
%If we want to use a list from the function:
shiftsY = randShift;
VCODE_mod = VCODE;

shiftsY = shiftsY/1000;  %convert mm to m

%VCODE_mod(1,3) = shiftsX(shift_selector);
VCODE_mod(1,4) = VCODE_mod(1,4)+shiftsY(randShift);
end
